simulink model "task4_simulink"  (R2024b)
settings: Solver=VariableStepAuto  StartTime=0.0  StopTime=100  RelTol=1e-3
values from neighbouring files (symbols this model uses):
  delta_trim = trim_solution(3)    [main.m]
  T_trim = trim_solution(1)    [main.m]
  x_trim = [ ... (first row only)    [main.m]
undefined symbols (not defined in the file or in its folder): params
settings Model: Creator=Admin  LastModifiedBy=Admin

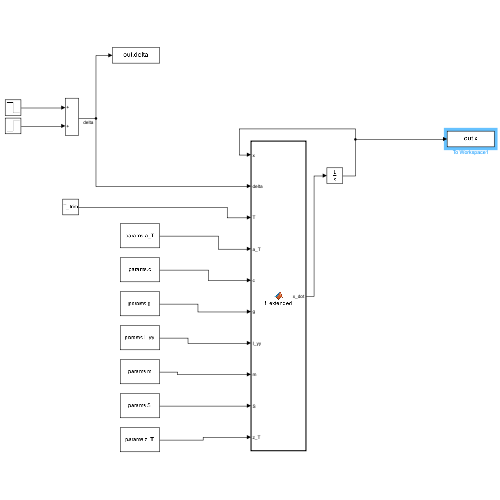
[thumbnail: Simulink's stored preview of the top-level diagram]
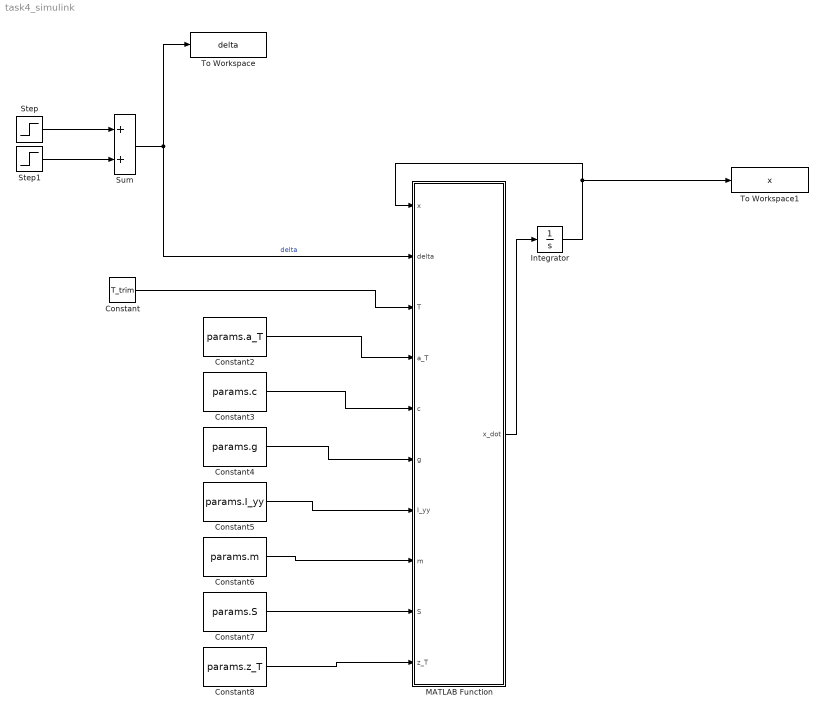
== system task4_simulink ==
  Constant : Constant  Value=T_trim
  Constant2 : Constant  Value=params.a_T
  Constant3 : Constant  Value=params.c
  Constant4 : Constant  Value=params.g
  Constant5 : Constant  Value=params.I_yy
  Constant6 : Constant  Value=params.m
  Constant7 : Constant  Value=params.S
  Constant8 : Constant  Value=params.z_T
  Integrator : Integrator  InitialCondition=x_trim
  MATLAB Function : MATLAB Function  TreatAsAtomicUnit=on
  Step : Step  Time=5  Before=delta_trim  After=delta_trim - pi/180  SampleTime=0
  Step1 : Step  Time=10  After=(pi/180)  SampleTime=0
  Sum : Sum
  To Workspace : ToWorkspace  VariableName=delta  SampleTime=-1
  To Workspace1 : ToWorkspace  VariableName=x  SaveFormat=Structure  SampleTime=-1
      settings: Save2DSignal=2-D array (concatenate along first dimension)
  wires:
  Step1/1 -> Sum/2
  Step/1 -> Sum/1
  Sum/1 -> To Workspace/1, MATLAB Function/2(delta)  "delta"
  MATLAB Function/1(x_dot) -> Integrator/1
  Integrator/1 -> To Workspace1/1, MATLAB Function/1(x)
  Constant/1 -> MATLAB Function/3(T)
  Constant2/1 -> MATLAB Function/4(a_T)
  Constant3/1 -> MATLAB Function/5(c)
  Constant4/1 -> MATLAB Function/6(g)
  Constant5/1 -> MATLAB Function/7(I_yy)
  Constant6/1 -> MATLAB Function/8(m)
  Constant7/1 -> MATLAB Function/9(S)
  Constant8/1 -> MATLAB Function/10(z_T)

== matlab function task4_simulink/MATLAB Function ==
  data: x input; delta input; T input; a_T input; c input; g input; I_yy input; m input; S input; z_T input; x_dot output
function x_dot = f_extended(x, delta, T, a_T, c, g, I_yy, m, S, z_T)
        u = x(1);
        w = x(2);
        q = x(3);
        theta = x(4);
        h = x(5);

        % delta = input(1);
        % T = input(2); % Thrust

        % [~, ~, ~, rho, ~, ~] = atmosisa(h);
        rho = 1.225;

        if (u ~= 0)
            alpha = atan(w / u);
        else
            alpha = 0;
        end

        V = sqrt(u ^ 2 + w ^ 2);

        c_L0 = 0.895;
        c_L_alpha = 5.01;
        c_L_delta = 0.722;
        c_D0 = 0.177;
        c_D_alpha = 0.232;
        c_D_alpha2 = 1.393;
        c_M0 = -0.046;
        c_M_alpha = -1.087;
        c_M_q = -7.055;
        c_M_delta = -1.88;

        c_L = @(alpha, delta) c_L0 + c_L_alpha * alpha + c_L_delta * delta;
        c_D = @(alpha) c_D0 + c_D_alpha * alpha + c_D_alpha2 * alpha ^ 2;
        c_M = @(alpha, delta, V, q) c_M0 + c_M_alpha * alpha + c_M_q * (c / V) * q + c_M_delta * delta;

        c_L = c_L(alpha, delta);
        c_D = c_D(alpha);
        c_M = c_M(alpha, delta, V, q);

        L = 0.5 * rho * V ^ 2 * S * c_L;
        D = 0.5 * rho * V ^ 2 * S * c_D;

        X_A = L * sin(alpha) - D * cos(alpha);
        Z_A = -L * cos(alpha) - D * sin(alpha);
        M_A = 0.5 * rho * V ^ 2 * S * c * c_M;

        X_T = T * cos(a_T);
        Z_T = -T * sin(a_T);
        M_T = T * z_T;

        u_dot = -q * w - g * sin(theta) + 1 / m * X_A + 1 / m * X_T;
        w_dot = q * u + g * cos(theta) + 1 / m * Z_A + 1 / m * Z_T;
        q_dot = 1 / I_yy * M_A + 1 / I_yy * M_T;
        theta_dot = q;
        h_dot = u * sin(theta) - w * cos(theta);

        x_dot = [u_dot; w_dot; q_dot; theta_dot; h_dot];
    end
